simulink model "Noa_Nofusion"  (R2020b)
settings: Solver=FixedStepDiscrete  StartTime=0.0  StopTime=Inf  FixedStep=0.01  RelTol=1e-3
PostLoadFcn:
  | if any(exist('dsrtsu_mdlpostloadfcn', 'file') ~= 0), dsrtsu_mdlpostloadfcn('Execute', bdroot); end
InitFcn:
  | , if any(exist('rtifpga_mdlclblib', 'file') ~= 0), rtifpga_mdlclblib('Init', bdroot); end,
  | , if any(exist('dsmpb_private', 'file') ~= 0), dsmpb_private('dsmpb_mdlclblib', 'Init', bdroot); end,
undefined symbols (not defined in the file or in its folder): ACC_TimeGap_DecSetSwt, ACC_TimeGap_IncSetSwt, AccelPedalPosn, AccelPedalPosnVldty, AccelPedlPosnDiagc, AccPedalOverride, ACU_ShiftInProgress, ADAS_Posn_CurLane, AESSwtReq, ALC_SwtReq, BrkPedalSts, CC_ACC_CANCEL_OFFSwt, CC_ACC_CRUISE_OFFSwt, CC_ACC_DecSetSpd_SetSwt, CC_ACC_IncSetSpd_ResuSwt, CC_ACCSwtErr, CharSpd_ms, CSA_NODE, CURRENT_GEAR, CurrentGearValid, DiscIntNeverNeededParam, DrvDoorSts, DrvSBR, DrvTrqReqOvld, ECMACCInterface, ECMRespACC, ELKSwtReq, EngLimpHomeSts, EngSpd, EngState, EngState_PHEV, EngTrqMaxActSpd, EngTrqMinAct, EPS_DrvInpTrqVal_HighReslolution, EPS_FailSts, EPS_LKATorqOvrlDlvd, EPS_LKATorqOvrlDlvdVld, EPS_LKATrqOvlDlvdSts, EPS_SteerMod, EPS_TrqSnsrSts, EQ4_APPINFO, EQ4_LA_ELEM, EQ4_LA_HDR, EQ4_LAP_ELEM, EQ4_LAP_HDR, EQ4_LH_ELEM, EQ4_LH_HDR, EQ4_LRE_ELEM, EQ4_LRE_HDR, ESS_PedSwtReq, ESS_VehSwtReq, FFogLmpSts_F_Pbox, FLWheelDriveDirection, FLWheelSpd, FrntWiprSwtSts, FrntWshrSwtSts, FRWheelDriveDirection, FRWheelSpd, HazardLmpSwtSts, HCU_AccelPedalPosn_Diag ... (+151)
libraries: simulink x144, dsmpblib x33, canfdmsglib x10
(part 15 of 20)

== matlab function Noa_Nofusion/TOS/Subsystem2/ACCOSM/HWA_Task100ms1/TargetSelect ==
  data: ACCmode input uint8 size=1; P0ID output uint8 size=1; vRef input single size=1; Valid input boolean size=15; Range input single size=15; Vr input single size=15; Dx input single size=15; Dy input single size=15; ArG input single size=15; Dyc input single size=15; Vyc input single size=15; Cnt input; plaus input single size=15; wCutIn input single size=15; spw input single size=15; spwLeft input single size=15; spwRight input single size=15; ReID input uint8 size=1; ReRange input single size=1; ReArG input single size=1; ReDx input single size=1; ReDy input single size=1; ReVx input single size=1; ReCutIn_b input boolean size=1; ReDyc input single size=1; ReVyc input single size=1; TargetLost_b input; tTargetLost input single size=1; dyLaneWidth input single size=1; Classfication input uint8 size=15; MoveSts input uint8 size=15; TarLimDx input single size=1; TarLimS0Dx input; TargetExistK1 input boolean size=1; P2ID output uint8 size=1; P3ID output uint8 size=1; P0Range output single size=1; P2Range output single size=1; P3Range output single size=1; P0Vr output single size=1; P2Vr output single size=1; P3Vr output single size=1; P0ArG output single size=1; P2ArG output single size=1; P3ArG output single size=1; P0Dx output single size=1; P2Dx output single size=1; P3Dx output single size=1; P0Dy output single size=1; P2Dy output single size=1; P3Dy output single size=1; TargetCutIn_b output boolean size=1; P0Dyc output single size=1; P0Vyc output single size=1; TargetExist output boolean size=1; TargetReplacedCntK1 input uint8; TargetReplacedCnt output uint8
function [P0ID,P2ID,P3ID,P0Range,P2Range,P3Range,P0Vr,P2Vr,P3Vr,P0ArG,P2ArG,P3ArG,...
    P0Dx,P2Dx,P3Dx,P0Dy,P2Dy,P3Dy,TargetCutIn_b,P0Dyc,P0Vyc,TargetExist,TargetReplacedCnt] = ...
    ATS(ACCmode,vRef,Valid,Range,Vr,Dx,Dy,ArG,Dyc,Vyc,Cnt,plaus,wCutIn,spw,spwLeft,spwRight,...
    ReID,ReRange,ReArG,ReDx,ReDy,ReVx,ReCutIn_b,ReDyc,ReVyc,TargetLost_b,tTargetLost,dyLaneWidth,...
    Classfication,MoveSts,TarLimDx,TarLimS0Dx,TargetExistK1,TargetReplacedCntK1)

% #codegen
% ACCMode
% 0x00:OFF mode
% 0x01:Passive mode(Reject)
% 0x02:Passive mode(Stand-by)
% 0x03:Active-Control mode
% 0x04:Brake-only mode
% 0x05:Override
% 0x06:Standstill
% 0x07:Failure mode
% 0x08~0x1F:Reserved

P0ID = uint8(0);
P2ID = uint8(0);
P3ID = uint8(0);
P0Range = single(255);
P2Range = single(255);
P3Range = single(255);
P0Vr = single(0);
P2Vr = single(0);
P3Vr = single(0);
P0ArG = single(0);
P2ArG = single(0);
P3ArG = single(0);
P0Dx = single(255);
P2Dx = single(255);
P3Dx = single(255);
P0Dy = single(0);
P2Dy = single(0);
P3Dy = single(0);
TargetExist = false;
TargetCutIn_b = false;
P0Dyc = single(0);
P0Vyc = single(0);

DycOffset = interpolate(single(50),single(0.35),single(80),single(0.6),ReDx);

if TargetLost_b
   TargetReplacedCnt = uint8(0);
else
   TargetReplacedCnt = min(uint8(255),TargetReplacedCntK1 + uint8(1));
end

if (ACCmode==1)||(ACCmode==2)||(ACCmode==3)||(ACCmode==4)||(ACCmode==5)||(ACCmode==6)||(ACCmode==9)
    if TargetExistK1==false   % first select target
        for i=1:15
            if (Valid(i)==1)&&(Cnt(i)>=3)&&...
                    (((vRef<=15.83)&&((MoveSts(i)==1)||(MoveSts(i)==2)||(MoveSts(i)==3)))||...
                    ((vRef>15.83)&&((MoveSts(i)==2)||(MoveSts(i)==3))))
                if (Classfication(i)==1)||(Classfication(i)==2)||(Classfication(i)==3)||(Classfication(i)==9)
                    if ((Range(i)<=TarLimS0Dx)&&(MoveSts(i)==1))||((Range(i)<=TarLimDx)&&((MoveSts(i)==2)||(MoveSts(i)==3)))
                        if (plaus(i)>=0.4)||((wCutIn(i)>0.7)&&(spw(i)>=0.8))||((spw(i)>0.95)&&(Range(i)<1.5*vRef))         % Need Check!
                            if Range(i)<P0Range
                                P0ID = uint8(i);
                                P0Range = Range(i);
                            end
                        else
                            if spwLeft(i)>0.2
                                if Range(i)<P2Range
                                    P2ID = uint8(i);
                                    P2Range = Range(i);
                                end
                            end
                            if spwRight(i)>0.2
                                if Range(i)<P3Range
                                    P3ID = uint8(i);
                                    P3Range = Range(i);
                                end
                            end
                        end
                    end
                end
            end
        end
    else
        k = ReID;
        if k<100        % No Target Lost!!!
            if (Valid(k)==0)
                for i=1:15
                    if (Valid(i)==1)&&...
                            (((vRef<=15.83)&&((MoveSts(i)==1)||(MoveSts(i)==2)||(MoveSts(i)==3)))||...
                            ((vRef>15.83)&&((MoveSts(i)==2)||(MoveSts(i)==3))))
                        if (Classfication(i)==1)||(Classfication(i)==2)||(Classfication(i)==3)||(Classfication(i)==9)
                            if ((Range(i)<=TarLimS0Dx)&&(MoveSts(i)==1))||((Range(i)<=TarLimDx)&&((MoveSts(i)==2)||(MoveSts(i)==3)))
                                if (plaus(i)>=0.4)||((wCutIn(i)>0.7)&&(spw(i)>=0.8))||((spw(i)>0.95)&&(Range(i)<1.5*vRef))
                                    if Range(i)<P0Range
                                        P0ID = uint8(i);
                                        P0Range = Range(i);
                                    end
                                else
                                    if spwLeft(i)>0.2
                                        if Range(i)<P2Range
                                            P2ID = uint8(i);
                                            P2Range = Range(i);
                                        end
                                    end
                                    if spwRight(i)>0.2
                                        if Range(i)<P3Range
                                            P3ID = uint8(i);
                                            P3Range = Range(i);
                                        end
                                    end
                                end
                            end
                        end
                    end
                end
            else
                temp = interpolate(single(5),single(10),single(30),single(20),vRef);
                
                if TargetReplacedCnt>4   % no Target lost  Or  After Target 4  cnt!
                    if ((Range(k)<=(TarLimS0Dx+temp))&&(MoveSts(k)==1))||((Range(k)<=(TarLimDx+temp))&&((MoveSts(k)==2)||(MoveSts(k)==3)))
                        if (plaus(k)>=0.2)||((wCutIn(k)>0.6)&&(spw(k)>=0.4))||(spw(k)>0.6)
                            if Range(k)<P0Range
                                P0ID = uint8(k);
                                P0Range = Range(k);
                            end
                        else
                            if spwLeft(k)>0.2
                                if Range(k)<P2Range
                                    P2ID = uint8(k);
                                    P2Range = Range(k);
                                end
                            end
                            if spwLeft(k)>0.2
                                if Range(k)<P3Range
                                    P3ID = uint8(k);
                                    P3Range = Range(k);
                                end
                            end
                        end
                    end
                else  % After lost Target  Replaced  1\2\3 Cnt ！
                    if (Range(k)<(TarLimDx+temp))
                        if (spw(k)>=0.8)||((wCutIn(k)>0.7)&&(spw(k)>=0.4))
                            if Range(k)<P0Range
                                P0ID = uint8(k);
                                P0Range = Range(k);
                            end
                        else
                            if spwLeft(k)>0.2
                                if Range(k)<P2Range
                                    P2ID = uint8(k);
                                    P2Range = Range(k);
                                end
                            end
                            if spwLeft(k)>0.2
                                if Range(k)<P3Range
                                    P3ID = uint8(k);
                                    P3Range = Range(k);
                                end
                            end
                        end
                    end
                end %  After lost Target Replaced  //end 
                for i=1:15
                    if (i~=k)&&(Valid(i)==1)&&...
                            (((vRef<=15.83)&&((MoveSts(i)==1)||(MoveSts(i)==2)||(MoveSts(i)==3)))||...
                            ((vRef>15.83)&&((MoveSts(i)==2)||(MoveSts(i)==3))))
                        if (Classfication(i)==1)||(Classfication(i)==2)||(Classfication(i)==3)||(Classfication(i)==9)
                            if ((Range(i)<=TarLimS0Dx)&&(MoveSts(i)==1))||((Range(i)<=TarLimDx)&&((MoveSts(i)==2)||(MoveSts(i)==3)))
                                if (plaus(i)>=0.4)||((wCutIn(i)>0.7)&&(spw(i)>=0.8))||((spw(i)>0.95)&&(Range(i)<1.5*vRef))
                                    if Range(i)<P0Range
                                        P0ID = uint8(i);
                                        P0Range = Range(i);
                                    end
                                else
                                    if spwLeft(i)>0.2
                                        if Range(i)<P2Range
                                            P2ID = uint8(i);
                                            P2Range = Range(i);
                                        end
                                    end
                                    if spwRight(i)>0.2
                                        if Range(i)<P3Range
                                            P3ID = uint8(i);
                                            P3Range = Range(i);
                                        end
                                    end
                                end
                            end
                        end
                    end
                end
            end
        else
            temp = interpolate(single(5),single(10),single(30),single(20),vRef);
            if (ReRange<(TarLimDx+temp))&&(tTargetLost<0.6)
                if (ReDyc<(DycOffset + dyLaneWidth))&&(ReDyc>(-dyLaneWidth - DycOffset))
                   P0ID = k;
                   P0Range = ReRange;
                end
            end
            for i=1:15
                if (Valid(i)==1)&&...
                        (((vRef<=15.83)&&((MoveSts(i)==1)||(MoveSts(i)==2)||(MoveSts(i)==3)))||...
                        ((vRef>15.83)&&((MoveSts(i)==2)||(MoveSts(i)==3))))
                    if (Classfication(i)==1)||(Classfication(i)==2)||(Classfication(i)==3)||(Classfication(i)==9)
                        if ((Range(i)<=TarLimS0Dx)&&(MoveSts(i)==1))||((Range(i)<=TarLimDx)&&((MoveSts(i)==2)||(MoveSts(i)==3)))
                            if (plaus(i)>=0.4)||((wCutIn(i)>0.7)&&(spw(i)>=0.8))||((spw(i)>0.95)&&(Range(i)<1.5*vRef))
                                if Range(i)<P0Range
                                    P0ID = uint8(i);
                                    P0Range = Range(i);
                                end
                            else
                                if spwLeft(i)>0.2
                                    if Range(i)<P2Range
                                        P2ID = uint8(i);
                                        P2Range = Range(i);
                                    end
                                end
                                if spwRight(i)>0.2
                                    if Range(i)<P3Range
                                        P3ID = uint8(i);
                                        P3Range = Range(i);
                                    end
                                end
                            end
                        end
                    end
                end
            end           
        end
    end
end

if (P0ID>0)&&(P0ID<100)
    TargetExist = true;
    P0Range = Range(P0ID);
    P0Vr = Vr(P0ID);
    P0ArG = ArG(P0ID);
    P0Dx = Dx(P0ID);
    P0Dy = Dy(P0ID);
    if wCutIn(P0ID)>0.6
       TargetCutIn_b = true;
    end
    P0Dyc = Dyc(P0ID);
    P0Vyc = Vyc(P0ID);
else
    if P0ID>100
        TargetExist = true;
        P0Range = ReRange;
        P0Vr = ReVx;
        P0ArG = ReArG;
        P0Dx = ReDx;
        P0Dy = ReDy;
        TargetCutIn_b = ReCutIn_b;
        P0Dyc = ReDyc;
        P0Vyc = ReVyc;
    end
end
if P2ID>0
    P2Range = Range(P2ID);
    P2Vr = Vr(P2ID);
    P2ArG = ArG(P2ID);
    P2Dx = Dx(P2ID);
    P2Dy = Dy(P2ID);
end
if P3ID>0
    P3Range = Range(P3ID);
    P3Vr = Vr(P3ID);
    P3ArG = ArG(P3ID);
    P3Dx = Dx(P3ID);
    P3Dy = Dy(P3ID);
end
end

== matlab function Noa_Nofusion/Chassis1/Subsystem/CheckSum8Bclc4 ==
  data: Data input; MsgByte output; DataID input
function MsgByte  = CheckSum8B(Data,DataID)
CRC_8_H1D_Tbl =[ 0x00, 0x1d, 0x3a, 0x27, 0x74, 0x69, 0x4e, 0x53, 0xe8, 0xf5, 0xd2, 0xcf, 0x9c, 0x81, 0xa6, 0xbb,...
    0xcd, 0xd0, 0xf7, 0xea, 0xb9, 0xa4, 0x83, 0x9e, 0x25, 0x38, 0x1f, 0x02, 0x51, 0x4c, 0x6b, 0x76, 0x87, 0x9a, 0xbd, 0xa0, 0xf3, 0xee, 0xc9, 0xd4,...
    0x6f, 0x72, 0x55, 0x48, 0x1b, 0x06, 0x21, 0x3c, 0x4a, 0x57, 0x70, 0x6d, 0x3e, 0x23, 0x04, 0x19, 0xa2, 0xbf, 0x98, 0x85, 0xd6, 0xcb, 0xec, 0xf1,...
    0x13, 0x0e, 0x29, 0x34, 0x67, 0x7a, 0x5d, 0x40, 0xfb, 0xe6, 0xc1, 0xdc, 0x8f, 0x92, 0xb5, 0xa8, 0xde, 0xc3, 0xe4, 0xf9, 0xaa, 0xb7, 0x90, 0x8d,...
    0x36, 0x2b, 0x0c, 0x11, 0x42, 0x5f, 0x78, 0x65, 0x94, 0x89, 0xae, 0xb3, 0xe0, 0xfd, 0xda, 0xc7, 0x7c, 0x61, 0x46, 0x5b, 0x08, 0x15, 0x32, 0x2f,...
    0x59, 0x44, 0x63, 0x7e, 0x2d, 0x30, 0x17, 0x0a, 0xb1, 0xac, 0x8b, 0x96, 0xc5, 0xd8, 0xff, 0xe2, 0x26, 0x3b, 0x1c, 0x01, 0x52, 0x4f, 0x68, 0x75,...
    0xce, 0xd3, 0xf4, 0xe9, 0xba, 0xa7, 0x80, 0x9d, 0xeb, 0xf6, 0xd1, 0xcc, 0x9f, 0x82, 0xa5, 0xb8, 0x03, 0x1e, 0x39, 0x24, 0x77, 0x6a, 0x4d, 0x50,...
    0xa1, 0xbc, 0x9b, 0x86, 0xd5, 0xc8, 0xef, 0xf2, 0x49, 0x54, 0x73, 0x6e, 0x3d, 0x20, 0x07, 0x1a, 0x6c, 0x71, 0x56, 0x4b, 0x18, 0x05, 0x22, 0x3f,...
    0x84, 0x99, 0xbe, 0xa3, 0xf0, 0xed, 0xca, 0xd7, 0x35, 0x28, 0x0f, 0x12, 0x41, 0x5c, 0x7b, 0x66, 0xdd, 0xc0, 0xe7, 0xfa, 0xa9, 0xb4, 0x93, 0x8e,...
    0xf8, 0xe5, 0xc2, 0xdf, 0x8c, 0x91, 0xb6, 0xab, 0x10, 0x0d, 0x2a, 0x37, 0x64, 0x79, 0x5e, 0x43, 0xb2, 0xaf, 0x88, 0x95, 0xc6, 0xdb, 0xfc, 0xe1,...
    0x5a, 0x47, 0x60, 0x7d, 0x2e, 0x33, 0x14, 0x09, 0x7f, 0x62, 0x45, 0x58, 0x0b, 0x16, 0x31, 0x2c, 0x97, 0x8a, 0xad, 0xb0, 0xe3, 0xfe, 0xd9, 0xc4];

CRC_temp=uint8(zeros(1));

for t_index = 1:2
    CRC_temp = bitxor(DataID(t_index),CRC_temp);
    CRC_temp = CRC_8_H1D_Tbl(CRC_temp+1);
end

for t_index = 10:16
    CRC_temp = bitxor(Data(t_index),CRC_temp);
    CRC_temp = CRC_8_H1D_Tbl(CRC_temp+1);
end
Data(9)=CRC_temp;
CRC_temp=uint8(zeros(1));
for t_index = 3:4
    CRC_temp = bitxor(DataID(t_index),CRC_temp);
    CRC_temp = CRC_8_H1D_Tbl(CRC_temp+1);
end

for t_index = 18:24
    CRC_temp = bitxor(Data(t_index),CRC_temp);
    CRC_temp = CRC_8_H1D_Tbl(CRC_temp+1);
end
Data(17)=CRC_temp;
MsgByte=Data;
end

== matlab function Noa_Nofusion/TOS/Subsystem2/ACCOSM/HWA_Task100ms1/TimeCalc ==
  data: SameTarget input boolean size=1; TargetID input uint8 size=1; tSameHandleTK1 input single size=1; tSameHandleT output single size=1
function tSameHandleT = TimeCalc(SameTarget,TargetID,tSameHandleTK1)

if TargetID~=0
    if SameTarget==true
        tSameHandleT = min(tSameHandleTK1 + single(0.1),single(1800));
    else
        tSameHandleT = single(0);
    end
else
    tSameHandleT = single(0);
end

== matlab function Noa_Nofusion/TOS/Subsystem2/ACCOSM/HWA_Task100ms1/Trajectory/Trajectory/AssignHighPriorityObjects ==
  data: ObjNumber input; TrajNumber input; BufNumber input; SlipDisLim input; ObjPrio input; ObjMatrix input; VxvRef input; ObjCntAlive input; ObjClass input; ObjDxv input; ObjDyv input; TrajUsedK1 input; TrajHistBufferBTrajEndK1 input; ObjTrajNumberK1 input; TrajCurrentIndexK1 input; TrajHistBufferBValidK1 input; TrajHistBufferDxvK1 input; TrajHistBufferDyvK1 input; TrajHistBufferTTimeStampK1 input; TrajHistBufferClassK1 input; TrajUsed output boolean; TrajHistBufferBTrajEnd output boolean; ObjTrajNumber output uint8; TrajCurrentIndex output uint8; TrajHistBufferBValid output boolean; TrajHistBufferDxv output single; TrajHistBufferDyv output single; TrajHistBufferTTimeStamp output single; TrajHistBufferClass output uint8
function [TrajUsed,TrajHistBufferBTrajEnd,ObjTrajNumber,TrajCurrentIndex,TrajHistBufferBValid,...
    TrajHistBufferDxv,TrajHistBufferDyv,...
    TrajHistBufferTTimeStamp,TrajHistBufferClass] = fcn(...
    ObjNumber,TrajNumber,BufNumber,SlipDisLim,ObjPrio,ObjMatrix,VxvRef,ObjCntAlive,ObjClass,ObjDxv,ObjDyv,...
    TrajUsedK1,TrajHistBufferBTrajEndK1,ObjTrajNumberK1,TrajCurrentIndexK1,...
    TrajHistBufferBValidK1,TrajHistBufferDxvK1,TrajHistBufferDyvK1,...
    TrajHistBufferTTimeStampK1,TrajHistBufferClassK1)

[TrajUsed,TrajHistBufferBTrajEnd,ObjTrajNumber,TrajCurrentIndex,TrajHistBufferBValid,...
    TrajHistBufferDxv,TrajHistBufferDyv,...
    TrajHistBufferTTimeStamp,TrajHistBufferClass] = Traj_AssignHighPriorityObjects(...
    ObjNumber,TrajNumber,BufNumber,SlipDisLim,ObjPrio,ObjMatrix,VxvRef,ObjCntAlive,ObjClass,ObjDxv,ObjDyv,...
    TrajUsedK1,TrajHistBufferBTrajEndK1,ObjTrajNumberK1,TrajCurrentIndexK1,...
    TrajHistBufferBValidK1,TrajHistBufferDxvK1,TrajHistBufferDyvK1,...
    TrajHistBufferTTimeStampK1,TrajHistBufferClassK1);
end

== matlab function Noa_Nofusion/TOS/Subsystem2/ACCOSM/HWA_Task100ms1/Trajectory/Trajectory/CalcCompensateEgoVehMove ==
  data: BufNumber input; TrajNumber input; tCycle input; dDeltaX input; dDeltaY input; CosOfPsi input; SinOfPsi input; TrajHistBufferBValidK1 input; TrajHistBufferDxvK1 input; TrajHistBufferDyvK1 input; TrajHistBufferBValid output; TrajHistBufferDxv output; TrajHistBufferDyv output; TrajHistBufferTTimeStampK1 input; TrajHistBufferTTimeStamp output
function [TrajHistBufferBValid,TrajHistBufferDxv,TrajHistBufferDyv,...
    TrajHistBufferTTimeStamp] = ...
    Compensate(BufNumber,TrajNumber,tCycle,dDeltaX,dDeltaY,CosOfPsi,SinOfPsi,...
    TrajHistBufferBValidK1,TrajHistBufferDxvK1,TrajHistBufferDyvK1,...
    TrajHistBufferTTimeStampK1)
%#codegen
TrajHistBufferBValid = TrajHistBufferBValidK1;
TrajHistBufferDxv = TrajHistBufferDxvK1;
TrajHistBufferDyv = TrajHistBufferDyvK1;
TrajHistBufferTTimeStamp = TrajHistBufferTTimeStampK1;

for i=1:TrajNumber
    for j=1:BufNumber
        if TrajHistBufferBValid(i,j)==true
            t_dx = TrajHistBufferDxv(i,j)-dDeltaX;
            t_dy = TrajHistBufferDyv(i,j)-dDeltaY;
            t_dxTmp = t_dx*CosOfPsi+t_dy*SinOfPsi;
            t_dyTmp = -t_dx*SinOfPsi+t_dy*CosOfPsi;
            if (t_dxTmp>-255)&&(t_dxTmp<255)&&(t_dyTmp>-255)&&(t_dyTmp<255)
                TrajHistBufferDxv(i,j) = t_dxTmp;
                TrajHistBufferDyv(i,j) = t_dyTmp;
            else
                TrajHistBufferBValid(i,j) = false;
            end
            
            TrajHistBufferTTimeStamp(i,j) = min(TrajHistBufferTTimeStamp(i,j)+tCycle,32);
            
            if TrajHistBufferDxv(i,j)<-1
                TrajHistBufferBValid(i,j) = false;
            end
        end
    end
end

== matlab function Noa_Nofusion/TOS/Subsystem2/ACCOSM/HWA_Task100ms1/Trajectory/Trajectory/CalcEgoVehMove ==
  data: dDeltaX output single size=1; tCycle input size=1; Kap input size=1; Vego input size=1; alpSideSlipAngle input size=1; dDeltaY output single size=1; CosOfPsi output single size=1; SinOfPsi output single size=1; WheelTrack input; SlipDislim output; Vch input
function [dDeltaX,dDeltaY,CosOfPsi,SinOfPsi,SlipDislim] = EgoVehicleMovement(tCycle,Kap,Vego,alpSideSlipAngle,WheelTrack,Vch)
%#codegen
if Kap==0
    dDeltaX = Vego*tCycle;
    dDeltaY = single(0);
    CosOfPsi = single(1);
    SinOfPsi = single(0);
    SlipDislim = Vch*1000;
else
    SlipDislim = max(WheelTrack*1000,min(tCycle*Vego,Kap*15));
    t_Psi = Kap*Vego*tCycle;
    SinOfPsi = sin(t_Psi);
    CosOfPsi = cos(t_Psi);
    t_dDeltaXTemp = SinOfPsi/Kap;
    t_dDeltaYTemp = 2*(sin(t_Psi/2)*sin(t_Psi/2))/Kap;
    dDeltaX = min(cos(alpSideSlipAngle)*t_dDeltaXTemp - sin(alpSideSlipAngle)*t_dDeltaYTemp,SlipDislim);
    dDeltaY = sin(alpSideSlipAngle)*t_dDeltaXTemp + cos(alpSideSlipAngle)*t_dDeltaYTemp;
end

== matlab function Noa_Nofusion/TOS/Subsystem2/ACCOSM/HWA_Task100ms1/Trajectory/Trajectory/Priority ==
  data: ObjNumber input; ObjValid input; ObjPrio output single; ObjClass input; ObjDx input; ObjMatrix output single
function [ObjPrio,ObjMatrix] = fcn(ObjNumber,ObjValid,ObjClass,ObjDx)
%#codegen
ObjPrio = single(zeros(15,1));

for i=1:ObjNumber
    if ObjValid(i)
        if ObjDx(i)<0
            ObjPrio(i)=single(0);
        else
            if (ObjClass(i)==2)||(ObjClass(i)==3)||(ObjClass(i)==5)
                t_ObjPrio=single(2*255);
            else
                t_ObjPrio=single(255);
            end
            ObjPrio(i) = t_ObjPrio - ObjDx(i);
        end
    else
        ObjPrio(i)=single(0);
    end
end

ObjMatrix=ObjPrio;

t_h=1;
while 1
    t_h = t_h*3+1;
    if t_h>=ObjNumber
        break;
    end
end

%   t_h = 121;
while 1
    t_h = fix(t_h/3);
    for i=(t_h+1):ObjNumber
        j=i;
        t_zw=ObjMatrix(i);
        while (j>t_h)&&(t_zw<ObjMatrix(j-t_h))
            ObjMatrix(j)=ObjMatrix(j-t_h);
            j=j-t_h;
        end
        ObjMatrix(j)=t_zw;
    end
    if t_h==1
        break;
    end
end

== matlab function Noa_Nofusion/TOS/Subsystem2/ACCOSM/HWA_Task100ms1/Trajectory/Trajectory/ReleaseLowPriorityObjects ==
  data: TrajUsed output; ObjNumber input; TrajNumber input; ObjPrio input; ObjMatrix input; ObjValid input; TrajCurrentIndex input; TrajUsedK1 input; TrajHistBufferBTrajEndK1 input; ObjTrajNumberK1 input; TrajHistBufferBTrajEnd output; ObjTrajNumber output
function [TrajUsed,TrajHistBufferBTrajEnd,ObjTrajNumber] =...
    fcn(ObjNumber,TrajNumber,ObjPrio,ObjMatrix,ObjValid,TrajCurrentIndex,...
    TrajUsedK1,TrajHistBufferBTrajEndK1,ObjTrajNumberK1)
%#codegen
TrajHistBufferBTrajEnd = TrajHistBufferBTrajEndK1;
TrajUsed = TrajUsedK1;
ObjTrajNumber = ObjTrajNumberK1;
ObjPrioLimit = ObjMatrix(ObjNumber-TrajNumber);

for i=1:ObjNumber
    if ObjValid(i)
        if (ObjPrio(i)==0)||(ObjPrio(i)<=ObjPrioLimit)
            j = ObjTrajNumber(i);
            if j<(TrajNumber+1)
                t = TrajCurrentIndex(j);
                TrajHistBufferBTrajEnd(j,t)=1;
                TrajUsed(j)=0;
                ObjTrajNumber(i)=255;
            end
        end
    end
end

== matlab function Noa_Nofusion/TOS/Subsystem2/ACCOSM/HWA_Task100ms1/Trajectory/Trajectory/StoreEgoTrajectory ==
  data: Pa output single; Pb output single; Pc output single; Pd output single; BufNumber input; tCycle input; EgoTrajHistCurrentIndex output uint8; EgoDDeltaX input; EgoDDeltaY input; EgoCosOfPsi input; EgoSinOfPsi input; EgoTrajHistDxv output; EgoTrajHistDyv output; EgoTrajHistTTimeStamp output; EgoTrajHistCurrentIndexK1 input; EgoTrajHistDxvK1 input single; EgoTrajHistDyvK1 input single; EgoTrajHistTTimeStampK1 input single
function [Pa,Pb,Pc,Pd,EgoTrajHistCurrentIndex,EgoTrajHistDxv,EgoTrajHistDyv,EgoTrajHistTTimeStamp]...
    = fcn(BufNumber,tCycle,EgoDDeltaX,EgoDDeltaY,EgoCosOfPsi,EgoSinOfPsi,...
    EgoTrajHistCurrentIndexK1,EgoTrajHistDxvK1,EgoTrajHistDyvK1,EgoTrajHistTTimeStampK1)
%#codegen
EgoTrajHistCurrentIndex = EgoTrajHistCurrentIndexK1;
EgoTrajHistDxv = EgoTrajHistDxvK1;
EgoTrajHistDyv = EgoTrajHistDyvK1;
EgoTrajHistTTimeStamp = EgoTrajHistTTimeStampK1;
% alpWheelAngleOffset = alpWheelAngleOffsetK1;

t_IdxActualElement = EgoTrajHistCurrentIndex;
if t_IdxActualElement==BufNumber
    t_IdxNextElement=uint8(1);
else
    t_IdxNextElement=t_IdxActualElement+1;
end

Temp1 = EgoTrajHistDxv(t_IdxActualElement) - EgoDDeltaX;
Temp2 = EgoTrajHistDyv(t_IdxActualElement) - EgoDDeltaY;
dDeltaS = Temp1*Temp1 + Temp2*Temp2;
t_AddPosition = ((EgoTrajHistTTimeStamp(t_IdxActualElement)+tCycle)>0.3);
t_AddPosition = t_AddPosition&(dDeltaS>4);
t_AddPosition = t_AddPosition|(dDeltaS>100);
for iBuf=1:BufNumber
    if (t_AddPosition==1)&&(iBuf==t_IdxNextElement)
        EgoTrajHistDxv(iBuf)=single(0);
        EgoTrajHistDyv(iBuf)=single(0);
        EgoTrajHistTTimeStamp(iBuf)=single(0);
        EgoTrajHistCurrentIndex = t_IdxNextElement;
    else
        dX = EgoTrajHistDxv(iBuf)-EgoDDeltaX;
        dY = EgoTrajHistDyv(iBuf)-EgoDDeltaY;
        if (EgoTrajHistDxv(iBuf)>-255)&&(dX>-255)&&(dX<255)&&(dY>-255)&&(dY<255)
            Temp1 = dX*EgoCosOfPsi + dY*EgoSinOfPsi;
            Temp2 = -dX*EgoSinOfPsi + dY*EgoCosOfPsi;
            if (Temp1>-255)&&(Temp1<255)&&(Temp2>-255)&&(Temp2<255)
                EgoTrajHistDxv(iBuf)=Temp1;
                EgoTrajHistDyv(iBuf)=Temp2;
                tDt = EgoTrajHistTTimeStamp(iBuf)+tCycle;
                if tDt>32
                    tDt=single(32);
                end
                EgoTrajHistTTimeStamp(iBuf) = tDt;
            else
                EgoTrajHistDxv(iBuf)=single(-255);
                EgoTrajHistDyv(iBuf)=single(-255);
                EgoTrajHistTTimeStamp(iBuf) = single(32);
            end
        else
            EgoTrajHistDxv(iBuf)=single(-255);
            EgoTrajHistDyv(iBuf)=single(-255);
            EgoTrajHistTTimeStamp(iBuf) = single(32);
        end
    end
end

t_Index = EgoTrajHistCurrentIndex;
t_Index1 = BufNumber + uint8(23);
t_Index2 = BufNumber + uint8(21);
t_Index3 = BufNumber + uint8(19);

if t_Index1>24
    t_Index1 = t_Index1 - uint8(24);
end
if t_Index2>24
    t_Index2 = t_Index2 - uint8(24);
end
if t_Index3>24
    t_Index3 = t_Index3 - uint8(24);
end

XiMa = [EgoTrajHistDxv(t_Index);EgoTrajHistDxv(t_Index1);EgoTrajHistDxv(t_Index2);EgoTrajHistDxv(t_Index3)];
YiMa = [EgoTrajHistDyv(t_Index);EgoTrajHistDyv(t_Index1);EgoTrajHistDyv(t_Index2);EgoTrajHistDyv(t_Index3)];

[Pa,Pb,Pc,Pd] = pl(XiMa,YiMa);

% if (abs(EgoTrajHistDyv(t_Index1))<0.1)&&(abs(EgoTrajHistDyv(t_Index2))<0.1)&&(abs(EgoTrajHistDyv(t_Index3))<0.1)
%     kapRef = 3*Pa*EgoTrajHistDxv(t_Index2) + 2*Pb;
%     AckConst = min((1+VxvRef*VxvRef/(26*26))*2.68/max(VxvRef,1),32767);
%     alpWheelAngleRef = VxvRef*kapRef*AckConst;
%     Raw = alpWheelAngleMean - alpWheelAngleRef;
%     if VxvRef>7.3
%         alpWheelAngleOffset = (Raw - alpWheelAngleOffset)/10000 + alpWheelAngleOffset;
%     end
% else
%     alpWheelAngleRef = single(255);
% end

== matlab function Noa_Nofusion/TOS/Subsystem2/ACCOSM/HWA_Task100ms1/VycCalc ==
  data: ObjVyc output single size=15; dxC0 input; aP0 input; bP0 input; aP1 input; bP1 input; ObjValid input boolean size=15; ObjDx input single size=15; ObjVxG input single size=15; ObjVyG input single size=15; ObjYawAngle output
function [ObjVyc,ObjYawAngle] = VycCalc(dxC0,aP0,bP0,aP1,bP1,ObjValid,ObjDx,ObjVxG,ObjVyG)

ObjVyc = single(zeros(15,1));
ObjYawAngle = single(zeros(15,1));

for i=1:15
    if ObjValid(i)
       t_dxv = ObjDx(i);
       t_VxG = ObjVxG(i);
       t_VyG = ObjVyG(i);
       
       if abs(t_VxG)<0.1
          if t_VyG>0.5
              ObjYawAngle(i) = single(1.57);
          end
          if t_VyG<-0.5
              ObjYawAngle(i) = single(-1.57);
          end
       else
           if t_VxG>0
               ObjYawAngle(i) = atan(t_VyG/t_VxG);
           else
               if t_VyG>0
                  ObjYawAngle(i) = single(3.1416) + atan(t_VyG/t_VxG);
               else
                  ObjYawAngle(i) = -single(3.1416) + atan(t_VyG/t_VxG);
               end
           end
       end
       
       t_bParabolaYNLane = single(1);
       if t_dxv<dxC0
          temp1 =  2*aP0*t_dxv + bP0;
          t_bParabolaXNLane = -temp1;
       else
          temp1 =  2*aP1*t_dxv + bP1;
          t_bParabolaXNLane = -temp1;
       end
       t_bParabolaMag = mag(t_bParabolaXNLane,t_bParabolaYNLane);
       t_bParabolaXNLane = t_bParabolaXNLane/t_bParabolaMag;
       t_bParabolaYNLane = t_bParabolaYNLane/t_bParabolaMag;
       temp1 = t_VxG*t_bParabolaXNLane;
       temp2 = t_VyG*t_bParabolaYNLane;
       
       ObjVyc(i) = temp1 + temp2;
    else
       ObjVyc(i) = single(0);
    end
end
end

function out = mag(x,y)
M = max(abs(x),abs(y));
N = min(abs(x),abs(y));
out = M + 0.322*N;
end

== matlab function Noa_Nofusion/TOS/Subsystem2/DOP/HWA_Task100ms1/OTL1/P0TrajHistCalc01 ==
  data: P0Dyc output; vRef input; tCycle input single; tSameHandle input single; CutIn input; P0Dx input single; P0Dy input single; P0TrajHistNum output uint8; EgoDDeltaX input single; EgoDDeltaY input single; EgoCosOfPsi input single; EgoSinOfPsi input single; TarLineValid input; TarLineA2 input; TarLineA1 input; TarLineA0 input; P0TrajHistDxv output single; P0TrajHistDyv output single; P0TrajHistNumK1 input uint8; P0TrajHistDxvK1 input single; P0TrajHistDyvK1 input single
function [P0Dyc,P0TrajHistNum,P0TrajHistDxv,P0TrajHistDyv]...
    = fcn(vRef, tCycle,tSameHandle,CutIn, P0Dx,P0Dy,EgoDDeltaX,EgoDDeltaY,EgoCosOfPsi,EgoSinOfPsi,...
    TarLineValid,TarLineA2,TarLineA1,TarLineA0,...
    P0TrajHistNumK1,P0TrajHistDxvK1,P0TrajHistDyvK1)
%#codegen
P0TrajHistNum = P0TrajHistNumK1;
P0TrajHistDxv = P0TrajHistDxvK1;
P0TrajHistDyv = P0TrajHistDyvK1;

if TarLineValid
    temp1 = TarLineA2*P0Dx*P0Dx + TarLineA1*P0Dx + TarLineA0;
    P0Dyc = P0Dy - temp1;
else
    P0Dyc = single(255);
end
                
if tSameHandle==0
    P0TrajHistNum = uint8(0);
    P0TrajHistDxv = single(zeros(24,1));
    P0TrajHistDyv = single(zeros(24,1));
else
    if tSameHandle==tCycle
        if (CutIn&&abs(P0Dyc)>0.5) || (abs(P0Dyc)>0.8)||(vRef>8)
            P0TrajHistDxv(1) = P0Dx;
            P0TrajHistDyv(1) = P0Dy;
            P0TrajHistNum = uint8(1);
        else
            P0TrajHistDxv(1) = P0Dx;
            P0TrajHistDyv(1) = P0Dy;
            P0TrajHistNum = uint8(1);
            
            if TarLineValid
                P0TrajHistDxv(2) = 0.6*P0Dx;
                temp2 = 0.36*TarLineA2*P0Dx*P0Dx + 0.6*TarLineA1*P0Dx + TarLineA0;
                P0TrajHistDyv(2) = P0Dyc + temp2;
                
                P0TrajHistDxv(3) = 0.3*P0Dx;
                temp3 = 0.09*TarLineA2*P0Dx*P0Dx + 0.3*TarLineA1*P0Dx + TarLineA0;
                P0TrajHistDyv(3) = P0Dyc + temp3;
                
                P0TrajHistDxv(4) = single(-1);
                temp4 = TarLineA2 - TarLineA1 + TarLineA0;
                P0TrajHistDyv(4) = P0Dyc + temp4;
                
                P0TrajHistNum = uint8(4);
            end
        end
    else
        Temp1 = P0TrajHistDxv(1) - EgoDDeltaX - P0Dx;
        Temp2 = P0TrajHistDyv(1) - EgoDDeltaY - P0Dy;
        dDeltaS = Temp1*Temp1 + Temp2*Temp2;
        
        t_d = interpolate(single(8),single(0.5),single(22),single(2.5),single(P0TrajHistNum));
        t_d = t_d*t_d;
        t_AddPosition = (dDeltaS>t_d);
        
        for iBuf=1:P0TrajHistNum
            dX = P0TrajHistDxv(iBuf)-EgoDDeltaX;
            dY = P0TrajHistDyv(iBuf)-EgoDDeltaY;
            P0TrajHistDxv(iBuf) = dX*EgoCosOfPsi + dY*EgoSinOfPsi;
            P0TrajHistDyv(iBuf) = -dX*EgoSinOfPsi + dY*EgoCosOfPsi;
            if (P0TrajHistDxv(iBuf)<-5)||(abs(P0TrajHistDyv(iBuf))>50)
                P0TrajHistNum = max(P0TrajHistNum - uint8(1),uint8(0));
            end
        end
        
        if t_AddPosition==true
            
            P0TrajHistNum = min(P0TrajHistNum + uint8(1),uint8(24));
            for iBuf= P0TrajHistNum:(-1):2
                P0TrajHistDxv(iBuf) = P0TrajHistDxv(iBuf-uint8(1));
                P0TrajHistDyv(iBuf) = P0TrajHistDyv(iBuf-uint8(1));
            end
            P0TrajHistDxv(1) = P0Dx;
            P0TrajHistDyv(1) = P0Dy;
        end
    end
end
end

function out = interpolate(x1,z1,x2,z2,Raw)
if Raw<=x1
    out = z1;
else
    if Raw>=x2
        out = z2;
    else
        out = z1 + (Raw-x1)*(z2-z1)/(x2-x1);
    end
end
end

== matlab function Noa_Nofusion/TOS/Subsystem2/DOP/HWA_Task100ms1/OTL1/P0TrajHistCalc1 ==
  data: P0TrajHistNum output uint8; P0TrajHistNum1 input uint8; P0TrajHistDxv1 input single; P0TrajHistDxv output single; P0TrajHistDyv1 input single; P0TrajHistDyv output single; LineValid output boolean; a output single; b output single; c output single; d output single; dxMin output single; dxMax output single
function [P0TrajHistNum,P0TrajHistDxv,P0TrajHistDyv,LineValid,a,b,c,d,dxMin,dxMax] = P0TrajHistMixCalc(...
    P0TrajHistNum1,P0TrajHistDxv1,P0TrajHistDyv1)

P0TrajHistDxv = single(zeros(48,1));
P0TrajHistDyv = single(zeros(48,1));
P0TrajHistNum = uint8(0);

if (P0TrajHistNum1>0)
    P0TrajHistDxv(1:P0TrajHistNum1) = P0TrajHistDxv1(1:P0TrajHistNum1);
    P0TrajHistDyv(1:P0TrajHistNum1) = P0TrajHistDyv1(1:P0TrajHistNum1);
    P0TrajHistNum = P0TrajHistNum1;
end

if P0TrajHistNum>=4
    dxMin = P0TrajHistDxv(P0TrajHistNum);
    dxMax = P0TrajHistDxv(1) + 6;
%     q2 = max(ceil(P0TrajHistNum/2),2);
%     q3 = max(ceil(P0TrajHistNum*3/4),3);
%     q4 = P0TrajHistNum;
%     MaX = [P0TrajHistDxv(1);P0TrajHistDxv(q2);P0TrajHistDxv(q3);P0TrajHistDxv(q4)];
%     MaY = [P0TrajHistDyv(1);P0TrajHistDyv(q2);P0TrajHistDyv(q3);P0TrajHistDyv(q4)];
%     [~,b,c,d] = pl(MaX,MaY);
    P = polyfit(P0TrajHistDxv(1:P0TrajHistNum),P0TrajHistDyv(1:P0TrajHistNum),2);
    b = P(1);
    c = P(2);
    d = P(3);

    a = single(0);
   LineValid = true;
   if dxMin>0.5
      LineValid = false; 
   end
else
   dxMin = single(0); 
   dxMax = single(0); 
   a = single(0);
   b = single(0);
   c = single(0);
   d = single(0);
   LineValid = false;
end

== matlab function Noa_Nofusion/TOS2/Subsystem1/ACCOSM/HWA_Task100ms1/ACC_DisplayBar ==
  data: TimeGap input; DisplayBar output uint8; DesireDistance input; ACCmode input; TargetRange input; Scale input; TargetExist input; DisplayBarK1 input uint8
function DisplayBar = fcn(TimeGap,DesireDistance,ACCmode,TargetRange,Scale,TargetExist,DisplayBarK1)
%#codegen
DisplayBar = DisplayBarK1;

ScaleDis = Scale*DesireDistance;
upScaleDis = (Scale+single(0.05))*DesireDistance;
lowScaleDis = (Scale-single(0.05))*DesireDistance;

i = TimeGap;

if (ACCmode==0)||(ACCmode==7)
    DisplayBar = uint8(0);
else
    if TargetExist==false
        DisplayBar=uint8(0);
    else
        switch(DisplayBarK1)
            case uint8(0)
                 if TargetRange> ScaleDis(i,3)
                     DisplayBar=uint8(4);
                 else
                     if TargetRange>ScaleDis(i,2)
                         DisplayBar=uint8(3);
                     else
                         if TargetRange>ScaleDis(i,1)
                             DisplayBar=uint8(2);
                         else
                             DisplayBar=uint8(1);
                         end
                     end
                 end
            case uint8(1)
                 if TargetRange> upScaleDis(i,3)
                     DisplayBar=uint8(4);
                 else
                     if TargetRange>upScaleDis(i,2)
                         DisplayBar=uint8(3);
                     else
                         if TargetRange>upScaleDis(i,1)
                             DisplayBar=uint8(2);
                         else
                             DisplayBar=uint8(1);
                         end
                     end
                 end
            case uint8(2)
                 if TargetRange> upScaleDis(i,3)
                     DisplayBar=uint8(4);
                 else
                     if TargetRange>upScaleDis(i,2)
                         DisplayBar=uint8(3);
                     else
                         if TargetRange>lowScaleDis(i,1)
                             DisplayBar=uint8(2);
                         else
                             DisplayBar=uint8(1);
                         end
                     end
                 end   
            case uint8(3)
                 if TargetRange> upScaleDis(i,3)
                     DisplayBar=uint8(4);
                 else
                     if TargetRange>lowScaleDis(i,2)
                         DisplayBar=uint8(3);
                     else
                         if TargetRange>lowScaleDis(i,1)
                             DisplayBar=uint8(2);
                         else
                             DisplayBar=uint8(1);
                         end
                     end
                end
            case uint8(4)
                 if TargetRange> lowScaleDis(i,3)
                     DisplayBar=uint8(4);
                 else
                     if TargetRange>lowScaleDis(i,2)
                         DisplayBar=uint8(3);
                     else
                         if TargetRange>lowScaleDis(i,1)
                             DisplayBar=uint8(2);
                         else
                             DisplayBar=uint8(1);
                         end
                     end
                 end      
        end    
    end
end

== matlab function Noa_Nofusion/TOS2/Subsystem1/ACCOSM/HWA_Task100ms1/Dyc ==
  data: kapTrajFiltK1 input single size=1; vRef input single size=1; kapTrajFilt output single size=1; kapCourseErr output single; kapTraj input single size=1; alpSideSlipAngle input single size=1; A2 input single size=1; A1 input single size=1; LineValid input boolean size=1; ObjDx input single size=15; ObjDy input single size=15; TarLineValid input boolean; TarLineA2 input single; TarLineA1 input single; TarLineA0 input single size=1; dxC0 output single size=1; aPC0 output single size=1; bPC0 output single size=1; cPC0 output single size=1; aPC1 output single size=1; bPC1 output single size=1; cPC1 output single size=1; ObjDyc output single size=15
function [kapTrajFilt,kapCourseErr,dxC0,aPC0,bPC0,cPC0,aPC1,bPC1,cPC1,ObjDyc] = ...
    DriveCourseCalc(kapTrajFiltK1,vRef,kapTraj,alpSideSlipAngle,...
    A2,A1,LineValid,ObjDx,ObjDy,TarLineValid,TarLineA2,TarLineA1,TarLineA0)

ObjDyc = single(zeros(15,1));

if vRef>8.33
    t_alpSideSlipAngle = -alpSideSlipAngle;
else
    t_alpSideSlipAngle = single(0);
end

temp1 = single(0.1)/(single(0.1) + interpolate(single(24),single(0),single(55),single(0.4),vRef));

kapTrajFilt = kapTrajFiltK1 + temp1*(kapTraj - kapTrajFiltK1);

temp1 = abs(kapTraj*vRef);

if (temp1<0.001)&&(vRef>8.3)
    t_kapTrajwHyst = single(0);
else
    t_kapTrajwHyst = kapTrajFilt;
end

if TarLineValid
    temp = interpolate(single(0.2),single(0.2),single(1.5),single(1),abs(TarLineA0));
    dxC0Min = single(3);
else
    temp = single(1);
    dxC0Min = single(10);
end

dxC0 = max(vRef*temp,dxC0Min);
aPC0 = 0.5*t_kapTrajwHyst*(single(1)+1.5*t_alpSideSlipAngle*t_alpSideSlipAngle);
bPC0 = t_alpSideSlipAngle;
cPC0 = single(0);

temp1 = single(0.1)*abs(t_kapTrajwHyst);
temp2 = min(single(0.00013),single(0.004)/max(vRef,single(10)));
kapCourseErr = max(temp1,temp2);

aPC1 = aPC0;
bPC1 = bPC0;
cPC1 = single(0);

Low = interpolate(single(4),single(1),single(20),single(0),abs(atan(A1)));    % low vehiclespeed lanechange Angle is 4deg~20deg;
High = interpolate(single(4),single(1),single(10),single(0),abs(atan(A1)));   % low vehiclespeed lanechange Angle is 4deg~10deg;
t_vRefFactor = interpolate(single(5),Low,single(25),High,vRef);

t_Factor = single(1)*t_vRefFactor;

if TarLineValid==true
    aPC1 = TarLineA2;
    bPC1 = TarLineA1;
    cPC1 = (aPC0 - aPC1)*dxC0*dxC0 + (bPC0 - bPC1)*dxC0;
else
    if LineValid
        aPC1 = aPC0*(1 - t_Factor) + A2*t_Factor;
        bPC1 = bPC0*(1 - t_Factor) + A1*t_Factor;
        cPC1 = (aPC0 - aPC1)*dxC0*dxC0 + (bPC0 - bPC1)*dxC0;
    end
end

for i=1:15
   if ObjDx(i)>dxC0
      ObjDyc(i) =  ObjDy(i) - (aPC1*ObjDx(i)*ObjDx(i) + bPC1*ObjDx(i) + cPC1);
   else
      ObjDyc(i) =  ObjDy(i) - (aPC0*ObjDx(i)*ObjDx(i) + bPC0*ObjDx(i));
   end
end
end


function out = interpolate(x1,z1,x2,z2,Raw)
if Raw<=x1
    out = z1;
else
    if Raw>=x2
        out = z2;
    else
        out = z1 + (Raw-x1)*(z2-z1)/(x2-x1);
    end
end
end

== matlab function Noa_Nofusion/TOS2/Subsystem1/ACCOSM/HWA_Task100ms1/DycCutIn ==
  data: ObjValid input boolean size=15; ObjDyc input single size=15; ObjMoveSts input uint8 size=15; ObjDycCutIn output single size=15; ObjMove_b output boolean size=15; ObjCnt input uint8 size=15; ObjDycHist input single size=15; ObjqDycHist input single size=15; dycFiltK1 input single size=15; ObjDycFilt output single size=15
function [ObjDycCutIn,ObjMove_b,ObjDycFilt] = ...
    ObjDycCutInCalc(ObjValid,ObjDyc,ObjMoveSts,ObjCnt,ObjDycHist,ObjqDycHist,dycFiltK1)
 
ObjDycCutIn = single(zeros(15,1));
ObjDycFilt = single(zeros(15,1));
ObjMove_b = false(15,1); 
 
for i=1:15
    if ObjValid(i)
        t_dyc = ObjDyc(i);
        t_dycHist = ObjDycHist(i);
        t_qDycHist = ObjqDycHist(i);
        
        weightDycHist = t_qDycHist*0.1;
        weightDyc = single(1) - weightDycHist;
        
        t_dycASI = weightDycHist*t_dycHist + weightDyc*t_dyc;
        ObjDycCutIn(i) = t_dycASI;
        
        if ObjCnt(i)>2
            ObjDycFilt(i) = 0.028*(t_dycASI - dycFiltK1(i)) + dycFiltK1(i);
        else
            ObjDycFilt(i) = t_dycASI;
        end
        if ObjMoveSts(i)==2
            ObjMove_b(i) = true;
        end
    end
end

== matlab function Noa_Nofusion/TOS2/Subsystem1/ACCOSM/HWA_Task100ms1/DycHistCalc ==
  data: TrajHistBufferBTrajEnd input boolean; ObjTrajNumber input uint8; ObjDycHist output single; TrajCurrentIndex input uint8; TrajHistBufferBValid input boolean; TrajHistBufferDxv input single; TrajHistBufferDyv input single; ObjValid input boolean; ObjqDycHist output single; dxC0 input; aP0 input; bP0 input; cP0 input; aP1 input; bP1 input; cP1 input
function [ObjDycHist,ObjqDycHist] = DycHistCalc(TrajHistBufferBTrajEnd,ObjTrajNumber,TrajCurrentIndex,...
    TrajHistBufferBValid,TrajHistBufferDxv,TrajHistBufferDyv,ObjValid,dxC0,aP0,bP0,cP0,aP1,bP1,cP1)

t_dxv = single(0);
t_dyv = single(0);
t_dxvK1 = single(0);
t_dyvK1 = single(0);
ObjDycHist = single(zeros(15,1));
ObjqDycHist = single(zeros(15,1));

for iObj=1:15
    t_TrajNumber = ObjTrajNumber(iObj);
    if t_TrajNumber<21
        t_End = false;
        t_Failed = false;
        t_TrajCurrentIndex = TrajCurrentIndex(t_TrajNumber);
        t_TrajEnd = TrajHistBufferBTrajEnd(t_TrajNumber,t_TrajCurrentIndex);
        if (ObjValid(iObj)==true)&&(t_TrajEnd==false)
            for k=1:24
                if t_End==false
                    if t_TrajCurrentIndex<k
                        t_Index = t_TrajCurrentIndex + uint8(25) - k;
                    else
                        t_Index = t_TrajCurrentIndex - k + uint8(1);
                    end
                    if t_Index==1
                        t_IndexK1 = uint8(24);
                    else
                        t_IndexK1 = t_Index - uint8(1);
                    end
                    t_ValidK1 = TrajHistBufferBValid(t_TrajNumber,t_IndexK1);
                    t_TrajEndK1 = TrajHistBufferBTrajEnd(t_TrajNumber,t_IndexK1);
                    t_dxv = TrajHistBufferDxv(t_TrajNumber,t_Index);
                    t_dxvK1 = TrajHistBufferDxv(t_TrajNumber,t_IndexK1);
                    t_dyv = TrajHistBufferDyv(t_TrajNumber,t_Index);
                    t_dyvK1 = TrajHistBufferDyv(t_TrajNumber,t_IndexK1);
                    
                    if (t_TrajEndK1==true)||(t_ValidK1==false)
                        t_End = true;
                        t_Failed = true;
                    end
                    if (t_dxv>=0)&&(t_dxvK1<=0)
                        t_End = true;
                    end
                end
            end
        end
        if (t_End==true)&&(t_Failed==false)
            if (t_dxv==t_dxvK1)
                t_dycHist = t_dyv;
            else
                t_dycHist = t_dyv - t_dxv*(t_dyvK1 - t_dyv)/(t_dxvK1 - t_dxv);
            end
            t_qDycHist = single(1);  
        else
            if (t_End==true)&&(t_Failed==true)&&(t_dxv>0)
                if t_dxv>(dxC0)
                    t_dycHist = t_dyv - (aP1*t_dxv*t_dxv + bP1*t_dxv + cP1); 
                else
                    t_dycHist = t_dyv - (aP0*t_dxv*t_dxv + bP0*t_dxv + cP0); 
                end
               t_qDycHist = max((single(80) - t_dxv)/single(80),single(0));
            else
                t_dycHist = single(0);
                t_qDycHist = single(0);
            end
        end
    else
        t_dycHist = single(0);
        t_qDycHist = single(0);
    end
    ObjDycHist(iObj) = t_dycHist;
    ObjqDycHist(iObj) = t_qDycHist;
end
